simulink model "TPS"  (R2022b)
settings: Solver=FixedStepDiscrete  StartTime=0.0  StopTime=10.0  RelTol=1e-3
settings Model: Creator=MAAM  LastModifiedBy=MAAM
settings OptimizationCC: DefaultParameterBehavior=Inlined  UseDivisionForNetSlopeComputation=on  GainParamInheritBuiltInType=on  UseFloatMulNetSlope=on  InlineInvariantSignals=on  PassReuseOutputArgsAs=Individual arguments  ZeroExternalMemoryAtStartup=off  ZeroInternalMemoryAtStartup=off  NoFixptDivByZeroProtection=on  EfficientFloat2IntCast=on  LifeSpan=1  OptimizeBlockOrder=speed  DifferentSizesBufferReuse=on  EfficientTunableParamExpr=on
settings DebuggingCC: ParameterTunabilityLossMsg=error
settings HardwareCC: ProdLongLongMode=on
settings SFSimCC: MATLABDynamicMemAlloc=off
settings RTWCC: Description=Embedded Coder  SystemTargetFile=ert.tlc  TemplateMakefile=ert_default_tmf  CreateSILPILBlock=SIL
settings CodeAppCC: ForceParamTrailComments=on  IgnoreCustomStorageClasses=off  OperatorAnnotations=on  SimulinkDataObjDesc=on  SFDataObjDesc=on  CustomSymbolStrGlobalVar=rt$N$M  CustomSymbolStrType=$N$M  CustomSymbolStrFcn=$N$M$F  CustomSymbolStrMacro=$N$M  InsertBlockDesc=on
settings ERTTargetCC: TargetLangStandard=C99 (ISO)  GenerateSampleERTMain=on  IncludeMdlTerminateFcn=off  CombineSignalStateStructs=on  SuppressErrorStatus=on  SupportAbsoluteTime=off  SupportComplex=off  InlinedParameterPlacement=NonHierarchical  ERTCustomFileTemplate=example_file_process.tlc  ERTFilePackagingFormat=CompactWithDataFile

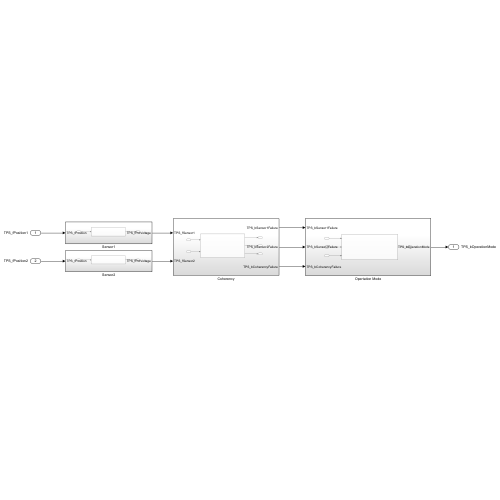
[thumbnail: Simulink's stored preview of the top-level diagram]
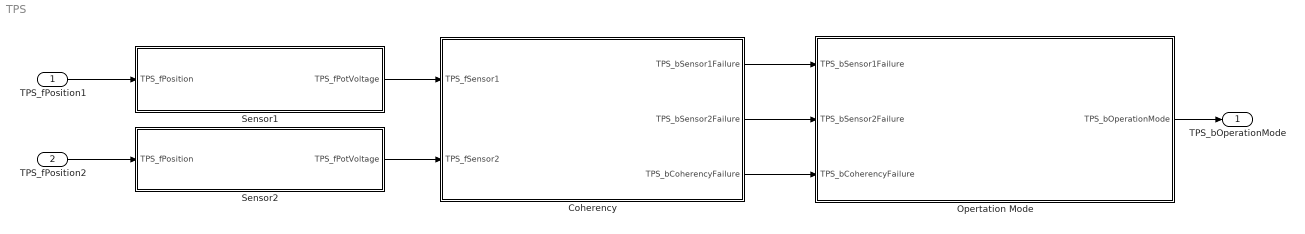
== system TPS ==
  TPS_fPosition1 : Inport  OutDataTypeStr=single
  TPS_fPosition2 : Inport  Port=2  OutDataTypeStr=single
  Coherency : Subsystem
  Opertation Mode : Subsystem
  Sensor1 : Subsystem
  Sensor2 : Subsystem
  TPS_bOperationMode : Outport  OutDataTypeStr=Enum: TPS_enuMode
  wires:
  Opertation Mode/1(TPS_bOperationMode) -> TPS_bOperationMode/1
  Coherency/1(TPS_bSensor1Failure) -> Opertation Mode/1(TPS_bSensor1Failure)
  Coherency/2(TPS_bSensor2Failure) -> Opertation Mode/2(TPS_bSensor2Failure)
  Coherency/3(TPS_bCoherencyFailure) -> Opertation Mode/3(TPS_bCoherencyFailure)
  TPS_fPosition1/1 -> Sensor1/1(TPS_fPosition)
  Sensor1/1(TPS_fPotVoltage) -> Coherency/1(TPS_fSensor1)
  TPS_fPosition2/1 -> Sensor2/1(TPS_fPosition)
  Sensor2/1(TPS_fPotVoltage) -> Coherency/2(TPS_fSensor2)

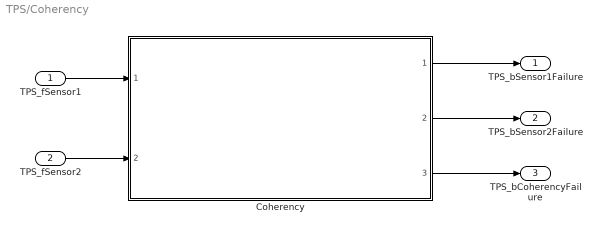
== system TPS/Coherency ==
  TPS_fSensor1 : Inport
  TPS_fSensor2 : Inport  Port=2
  Coherency : Subsystem  TreatAsAtomicUnit=on  ReferencedSubsystem=TPSC  Max=4.5  Min=0.5
  TPS_bSensor1Failure : Outport
  TPS_bSensor2Failure : Outport  Port=2
  TPS_bCoherencyFailure : Outport  Port=3
  wires:
  Coherency/1 -> TPS_bSensor1Failure/1
  TPS_fSensor1/1 -> Coherency/1
  TPS_fSensor2/1 -> Coherency/2
  Coherency/3 -> TPS_bCoherencyFailure/1
  Coherency/2 -> TPS_bSensor2Failure/1

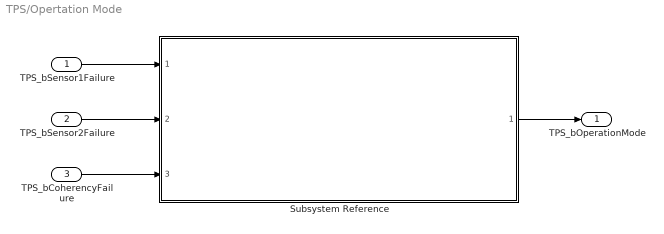
== system TPS/Opertation Mode ==
  TPS_bSensor1Failure : Inport
  TPS_bSensor2Failure : Inport  Port=2
  TPS_bCoherencyFailure : Inport  Port=3
  Subsystem Reference : Subsystem  ReferencedSubsystem=TPSM
  TPS_bOperationMode : Outport
  wires:
  TPS_bCoherencyFailure/1 -> Subsystem Reference/3
  TPS_bSensor2Failure/1 -> Subsystem Reference/2
  TPS_bSensor1Failure/1 -> Subsystem Reference/1
  Subsystem Reference/1 -> TPS_bOperationMode/1

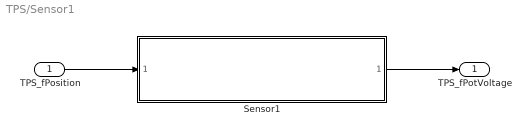
== system TPS/Sensor1 ==
  TPS_fPosition : Inport
  Sensor1 : Subsystem  TreatAsAtomicUnit=on  ReferencedSubsystem=TPSS  Max=4.5  Min=0.5
  TPS_fPotVoltage : Outport
  wires:
  Sensor1/1 -> TPS_fPotVoltage/1
  TPS_fPosition/1 -> Sensor1/1

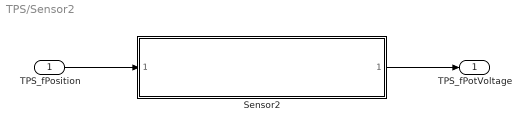
== system TPS/Sensor2 ==
  TPS_fPosition : Inport
  Sensor2 : Subsystem  TreatAsAtomicUnit=on  ReferencedSubsystem=TPSS  Max=0.5  Min=4.5
  TPS_fPotVoltage : Outport
  wires:
  Sensor2/1 -> TPS_fPotVoltage/1
  TPS_fPosition/1 -> Sensor2/1
